simulink model "PMSM_ESO"  (R2023b)
settings: Solver=ode4  StartTime=0.0  StopTime=0.8  FixedStep=2e-6  RelTol=1e-3
settings Model: Creator=Y  LastModifiedBy=Y

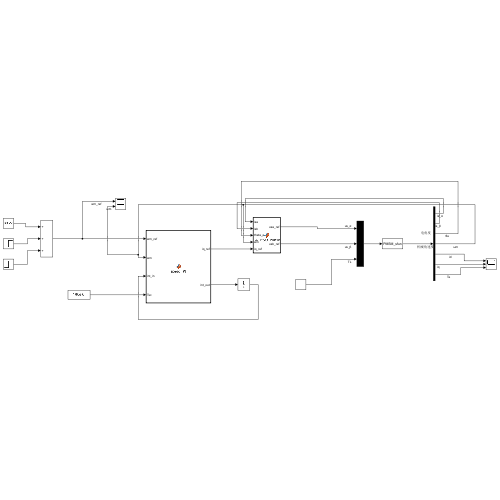
[thumbnail: Simulink's stored preview of the top-level diagram]
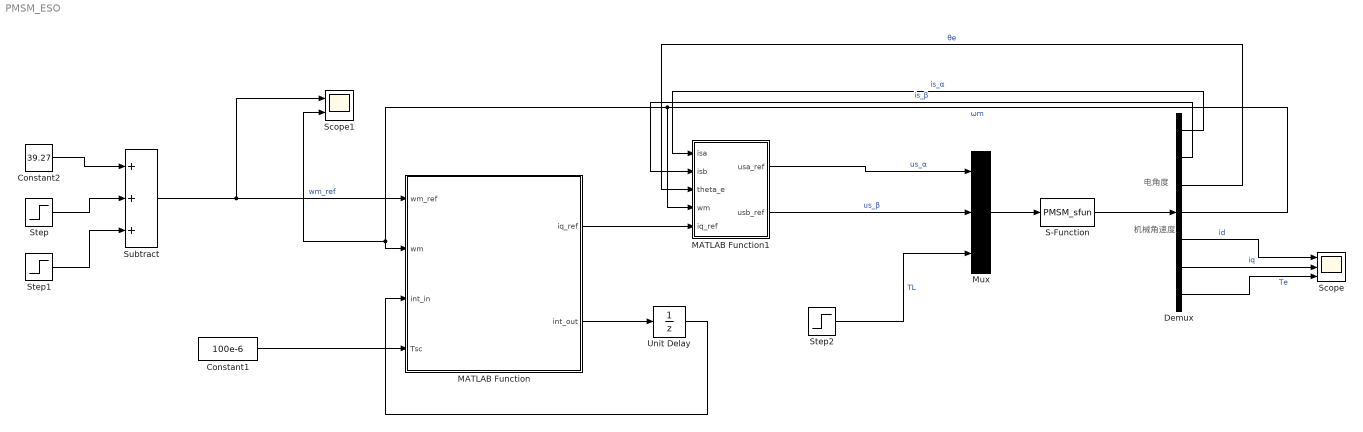
== system PMSM_ESO ==
  note: 机械角速度
  note: 电角度
  Constant1 : Constant  Value=100e-6
  Constant2 : Constant  Value=39.27
  Demux : Demux  Outputs=7
  MATLAB Function : MATLAB Function  TreatAsAtomicUnit=on
  MATLAB Function1 : MATLAB Function  TreatAsAtomicUnit=on
  Mux : Mux  Inputs=3
  S-Function : S-Function  FunctionName=PMSM_sfun  SFunctionDeploymentMode=off  EnableBusSupport=off
  Scope : Scope  NumInputPorts=3
  Scope1 : Scope  NumInputPorts=2
  Step : Step  Time=0.1  After=39.27  SampleTime=0
  Step1 : Step  Time=0.5  After=78.54  SampleTime=0
  Step2 : Step  Time=0.3  After=10  SampleTime=0
  Subtract : Sum  Inputs=+++
  Unit Delay : UnitDelay  SampleTime=-1  HasFrameUpgradeWarning=on
  wires:
  MATLAB Function/2(int_out) -> Unit Delay/1
  Unit Delay/1 -> MATLAB Function/3(int_in)
  MATLAB Function/1(iq_ref) -> MATLAB Function1/5(iq_ref)
  S-Function/1 -> Demux/1
  Demux/1 -> MATLAB Function1/1(isa)  "is_α"
  Demux/2 -> MATLAB Function1/2(isb)  "is_β"
  Demux/3 -> MATLAB Function1/3(theta_e)  "θe"
  Demux/4 -> MATLAB Function1/4(wm), Scope1/2, MATLAB Function/2(wm)  "ωm"
  Demux/5 -> Scope/1  "id"
  Demux/7 -> Scope/3  "Te"
  Mux/1 -> S-Function/1
  MATLAB Function1/1(usa_ref) -> Mux/1  "us_α"
  MATLAB Function1/2(usb_ref) -> Mux/2  "us_β"
  Step2/1 -> Mux/3  "TL"
  Constant1/1 -> MATLAB Function/4(Tsc)
  Constant2/1 -> Subtract/1
  Step/1 -> Subtract/2
  Step1/1 -> Subtract/3
  Demux/6 -> Scope/2  "iq"
  Subtract/1 -> Scope1/1, MATLAB Function/1(wm_ref)  "wm_ref"

== matlab function PMSM_ESO/MATLAB Function1 ==
  settings: updateMethod=DISCRETE  sampleTime=100e-6
  data: isa input; usa_ref output; isb input; theta_e input; wm input; iq_ref input; usb_ref output
function [usa_ref, usb_ref] = MFPCC_ESO_PMSM_fcn(isa, isb, theta_e, wm, iq_ref)
% MFPCC+ESO 控制器（αβ 坐标系）
% 输入：isa, isb（αβ 电流测量值），theta_e, wm（电角度、转速），iq_ref（速度环输出）
% 输出：usa_ref, usb_ref（αβ 参考电压，连续矢量）

% --- 电机参数（仅用于电压限幅，控制器本身不用）---
Udc = 540;
Np  = 4;

% --- MFPCC 参数（论文 Table I）---
Tsc = 100e-6;
alpha = 50;

% --- ESO 参数（论文 Section IV-B）---
omega0 = 8500;
beta1  = 2 * omega0;
beta2  = omega0^2;
beta01 = Tsc * beta1;
beta02 = Tsc * beta2;

% --- persistent 变量（ESO 状态，跨步保持）---
persistent is_hat F_hat us_prev spd_int
if isempty(is_hat)
    is_hat  = [0; 0];
    F_hat   = [0; 0];
    us_prev = [0; 0];
    spd_int = 0;
end

% --- 电流参考：dq → αβ，考虑一步延迟补偿（论文式21）---
id_ref = 0;
we = Np * wm;
theta_k2 = theta_e + 2 * we * Tsc;
is_ref_a = id_ref * cos(theta_k2) - iq_ref * sin(theta_k2);
is_ref_b = id_ref * sin(theta_k2) + iq_ref * cos(theta_k2);

% --- ESO 更新（论文式13）---
is_meas = [isa; isb];
err = is_hat - is_meas;
is_hat_next = is_hat + Tsc * (F_hat + alpha * us_prev) - beta01 * err;  % k+1时刻
F_hat_next  = F_hat - beta02 * err;

% --- MFPCC 控制律（论文式20）---
is_ref_k2 = [is_ref_a; is_ref_b];% k+2时刻
us_ref = (is_ref_k2 - is_hat_next) / (alpha * Tsc) - F_hat_next / alpha;

% --- 电压限幅 ---
Us_max = Udc / sqrt(3);
us_mag = sqrt(us_ref(1)^2 + us_ref(2)^2);
if us_mag > Us_max
    us_ref = us_ref * (Us_max / us_mag);
end

% --- 更新 persistent 状态 ---
is_hat  = is_hat_next;
F_hat   = F_hat_next;
us_prev = us_ref;

% --- 输出 ---
usa_ref = us_ref(1);
usb_ref = us_ref(2);
end

== matlab function PMSM_ESO/MATLAB Function ==
  settings: updateMethod=DISCRETE  sampleTime=100e-6
  data: wm_ref input; iq_ref output; wm input; int_in input; Tsc input; int_out output
function [iq_ref, int_out] = speed_PI(wm_ref, wm, int_in, Tsc)
% 速度环 PI 控制器
% 输入：wm_ref（参考转速），wm（实际转速），int_in（积分项），Tsc（控制周期）
% 输出：iq_ref（q轴电流参考），int_out（更新后积分项）

Kp = 2.0;
Ki = 50;
iq_max = 8.2;   % 2倍额定电流

wm_err = wm_ref - wm;
int_out = int_in + Ki * wm_err * Tsc;
iq_ref = Kp * wm_err + int_out;

% 限幅 + 抗饱和
if iq_ref > iq_max
    iq_ref = iq_max;
    int_out = int_in;  % 回退积分
elseif iq_ref < -iq_max
    iq_ref = -iq_max;
    int_out = int_in;
end
end
